simulink library "cft"  (Simulink 8.1)
settings: Solver=ode1  StartTime=0.0  StopTime=Inf  FixedStep=0.001  RelTol=1e-3
PostLoadFcn:
  | , if any(exist('dsrtsu_mdlpostloadfcn', 'file') == [2, 3, 6]), try dsrtsu_mdlpostloadfcn('Execute', bdroot); catch fprintf('Error in PostLoadFcn (dsrtsu_mdlpostloadfcn) for model "%s":\n %s\n', bdroot, lasterr); end, end,
undefined symbols (not defined in the file or in its folder): FALSE, KJUD_ACCFollowMErrorGParam_num, KJUD_ACCFollowMFFParam_num, KJUD_ACCFollowMInitialIParam_num, KJUD_ACCFollowMKdParam_num, KJUD_ACCFollowMKiParam_num, KJUD_ACCFollowMKpParam_num, KJUD_ACCFollowMMaxIParam_num, KJUD_ACCFollowMMinIParam_num, KJUD_ACCFollowMResetIParam_num
libraries: hcu_lib x1
settings Model: DSRTSU_INTERNAL_RTI_VER=450  DSRTSU_INTERNAL_RTI_TYPE=rti1401  RTICANMMDATA=struct('GeneralSetupData',struct('modelroot','D:\Projects\ELN150201\Repositories\Taiwan\trunk\AdasDragon\software\sw_development\arch\app\jud','generalsettings',struct('filesettings',struct('destfolder',struct('Name','RTICANMM_FILES','Check',1),'buildfolder',struct('Name','.','Check',1),'AbsDestfolder',struct('Name','D:\Projects\ELN150201\Repositories\Taiwan\trunk\AdasDragon\software\sw_development\arch\app\jud\RTICANMM_FILES'),'AbsBuildfolder',struct('Name','D:\Projects\ELN150201\Repositories\Taiwan\trunk\AdasDragon\software\sw_development\arch\app\jud'))),'options',struct('addpaths',1,'rmpaths',1,'addtrcexclusion',logical(1),'cannavigator',struct('checkmonitoring',0),'show_usrtrc',0,'use_usrtrc',0),'advanced',struct('options',[1 1 1 1 1 1 1 1 1 1 1 1 1 1 1 1 1 1 1 1 1 1 1 1 1 1 1 1 1 1 1 1 1 1 1 1 1 1 1 1 1 1 1 1 1 1 1 1 1 1 1 1 1 1 1 1 1 1 1 1 1 1 1 1 1 1 1 1 1 1 1 1 1 1 1 1 1 1 1 1 1 1 1 1 1 1 1 1 1 1 1 1 1 1 1 1 1 1 1 1]),'MPSetup',{{}},'modelname','cft','block','cft'))  DSRTSU_INTERNAL_RTIFPGA=40  Creator=AT015411  LastModifiedBy=AT015086

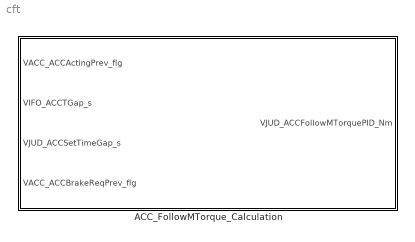
== system cft ==
  ACC_FollowMTorque_Calculation : Subsystem

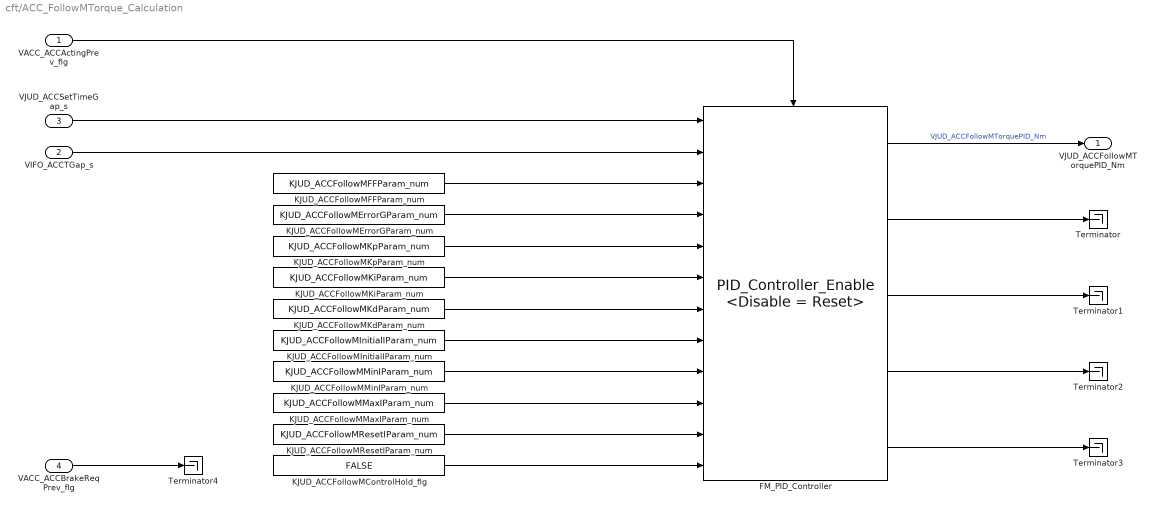
== system cft/ACC_FollowMTorque_Calculation ==
  VACC_ACCActingPrev_flg : Inport
  VIFO_ACCTGap_s : Inport  Port=2
  VJUD_ACCSetTimeGap_s : Inport  Port=3
  VACC_ACCBrakeReqPrev_flg : Inport  Port=4
  FM_PID_Controller : hcu_lib/PID_Controller_Enable <Disable = Reset>  SystemSampleTime=-1
  KJUD_ACCFollowMControlHold_flg : Constant  Value=FALSE  OutDataTypeStr=boolean
  KJUD_ACCFollowMErrorGParam_num : Constant  Value=KJUD_ACCFollowMErrorGParam_num
  KJUD_ACCFollowMFFParam_num : Constant  Value=KJUD_ACCFollowMFFParam_num
  KJUD_ACCFollowMInitialIParam_num : Constant  Value=KJUD_ACCFollowMInitialIParam_num
  KJUD_ACCFollowMKdParam_num : Constant  Value=KJUD_ACCFollowMKdParam_num
  KJUD_ACCFollowMKiParam_num : Constant  Value=KJUD_ACCFollowMKiParam_num
  KJUD_ACCFollowMKpParam_num : Constant  Value=KJUD_ACCFollowMKpParam_num
  KJUD_ACCFollowMMaxIParam_num : Constant  Value=KJUD_ACCFollowMMaxIParam_num
  KJUD_ACCFollowMMinIParam_num : Constant  Value=KJUD_ACCFollowMMinIParam_num
  KJUD_ACCFollowMResetIParam_num : Constant  Value=KJUD_ACCFollowMResetIParam_num
  Terminator{,1..4} (5 alike) : Terminator
  VJUD_ACCFollowMTorquePID_Nm : Outport
  wires:
  VJUD_ACCSetTimeGap_s/1 -> FM_PID_Controller/1
  FM_PID_Controller/1 -> VJUD_ACCFollowMTorquePID_Nm/1  "VJUD_ACCFollowMTorquePID_Nm"
  KJUD_ACCFollowMKpParam_num/1 -> FM_PID_Controller/5
  KJUD_ACCFollowMKiParam_num/1 -> FM_PID_Controller/6
  KJUD_ACCFollowMKdParam_num/1 -> FM_PID_Controller/7
  KJUD_ACCFollowMInitialIParam_num/1 -> FM_PID_Controller/8
  KJUD_ACCFollowMResetIParam_num/1 -> FM_PID_Controller/11
  KJUD_ACCFollowMMaxIParam_num/1 -> FM_PID_Controller/10
  KJUD_ACCFollowMMinIParam_num/1 -> FM_PID_Controller/9
  KJUD_ACCFollowMFFParam_num/1 -> FM_PID_Controller/3
  KJUD_ACCFollowMErrorGParam_num/1 -> FM_PID_Controller/4
  VACC_ACCActingPrev_flg/1 -> FM_PID_Controller/Enable
  VACC_ACCBrakeReqPrev_flg/1 -> Terminator4/1
  FM_PID_Controller/2 -> Terminator/1
  FM_PID_Controller/3 -> Terminator1/1
  FM_PID_Controller/4 -> Terminator2/1
  FM_PID_Controller/5 -> Terminator3/1
  VIFO_ACCTGap_s/1 -> FM_PID_Controller/2
  KJUD_ACCFollowMControlHold_flg/1 -> FM_PID_Controller/12
